simulink model "sampleModel2089"  (R2023a)
settings: Solver=VariableStepAuto  StartTime=0.0  StopTime=10.0  RelTol=1e-3
libraries: hdlsllib x3, simulink x3
settings Model: Creator=user1  LastModifiedBy=user1

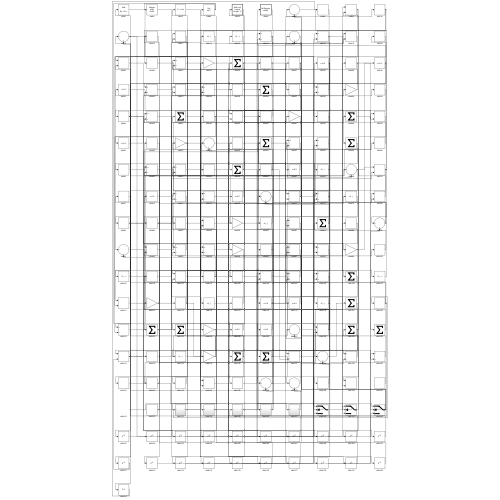
[thumbnail: Simulink's stored preview of the top-level diagram]
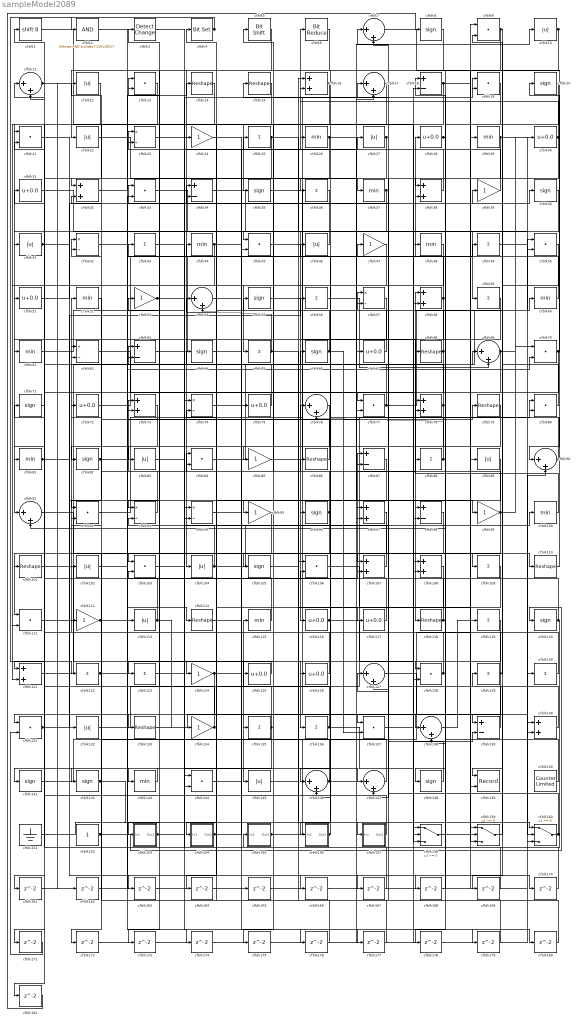
== system sampleModel2089 ==
  cfblk1 : ArithShift  BitShiftNumber=8
  cfblk{10,12,22,27,41,46,83,89,102,104,113,132,145} (13 alike) : Abs  SaturateOnIntegerOverflow=off
  cfblk{26,29,37,44,48,52,60..61,81,100,115,143} (12 alike) : MinMax
  cfblk{14..15,68,79,86,101,110,114,118,133} (10 alike) : Reshape
  cfblk{9,13,19,21,33,45,50,70,77,80,84,92,103,106,111,128,131,137,144} (19 alike) : DotProduct  OutDataTypeStr=Inherit: Inherit via internal rule
  cfblk{8,20,35,40,55,64,66,71,82,96,105,120,141..142,148} (15 alike) : Signum
  cfblk{16,32,38,58,73,78,97,107..108,121,140} (11 alike) : Sum
  cfblk{25,36,43,49,56,59,65,88,109,119,122..123,129..130,135..136} (16 alike) : Sum  Inputs=+
  cfblk{7,11,17,54,69,76,90..91,127,138,146..147} (12 alike) : Sum  Inputs=|++
  cfblk{24,39,47,53,85,95,99,112,124,134} (10 alike) : Gain
  cfblk{28,30..31,51,67,72,75,116..117,125..126} (11 alike) : Bias  Bias=0.0  SaturateOnIntegerOverflow=off
  cfblk{18,34,63,87,98,139} (6 alike) : Sum  Inputs=+-
  cfblk149 : Record  FileSettingsInternal="{\"entries\":[{\"content\":{\"excelSettings\":{\"content\":{},\"type\":\"Streamout.ExcelSettings\"}},\"type\":\"Streamout.FileSettingStorage\",\"uuid\":\"\"}],\"packageUris\":[\"http:\\/\\/schema.mathworks.com\\/mf0\\/streamout_blocks\\/R2020a\"],\"version\":\"1.0\"}"  Layout=[1 1]  SignalsInternal="{\"entries\":[{\"content\":{\"signals\":[{\"content\":{\"blockPath\":[],\"dimensions\":[1],\"domain\":\"\",\"lineColor\":\"#a2142f\",\"plots\":[1],\"port\":1,\"signalID\":6674,\"signalName\":\"XY Graph:1\"},\"type\":\"RecordBlkView.Signal\",\"uuid\":\"\"},{\"content\":{\"blockPath\":[],\"dimensions\":[1],\"domain\":\"\",\"lineColor\":\"#139fff\",\"plots\":[1],\"port\":2,\"signalID\":6677,\"signalName\":\"XY Graph:2\"},\"type\":\"RecordBlkView.Signal\",\"uuid\":\"\"}]},\"type\":\"RecordBlkView.InputSignals\",\"uuid\":\"\"}],\"packageUris\":[\"http:\\/\\/schema.mathworks.com\\/mf0\\/streamout_blocks\\/R2020a\"],\"version\":\"1.0\"}"  VisualizationBindings="{\"xyplotplugin\":{\"info\":[{\"series\":[{\"bindingParametersList\":[{\"parameter\":\"X-Axis\",\"signalID\":6674,\"signalName\":\"XY Graph:1\"},{\"parameter\":\"Y-Axis\",\"signalID\":6677,\"signalName\":\"XY Graph:2\"}],\"seriesID\":29365}],\"subplotID\":1}]}}"  CompatibilityTag=XY  st=-1
  cfblk150 : hdlsllib/Sources/Counter Limited  uplimit=7  tsamp=-1
  cfblk151 : Ground
  cfblk152 : Constant  SampleTime=-1
  cfblk153 : Subsystem
      settings: LibrarySourceBlock=|
      | hdlsllib/Ports &
      | Subsystems/Subsystem
  cfblk154 : Subsystem
      settings: LibrarySourceBlock=|
      | hdlsllib/Ports &
      | Subsystems/Subsystem
  cfblk155 : Subsystem
      settings: LibrarySourceBlock=|
      | hdlsllib/Ports &
      | Subsystems/Subsystem
  cfblk156 : Subsystem
      settings: LibrarySourceBlock=|
      | hdlsllib/Ports &
      | Subsystems/Subsystem
  cfblk157 : Subsystem
      settings: LibrarySourceBlock=|
      | hdlsllib/Ports &
      | Subsystems/Subsystem
  cfblk158 : Switch  SaturateOnIntegerOverflow=off  InputSameDT=off
  cfblk159 : Switch  SaturateOnIntegerOverflow=off  InputSameDT=off
  cfblk160 : Switch  SaturateOnIntegerOverflow=off  InputSameDT=off
  cfblk{161..181} (21 alike) : Delay  SampleTime=1
  cfblk2 : simulink/Logic and Bit Operations/Bitwise Operator  logicop=AND  UseBitMask=on  BitMask=bin2dec('11011001')  BitMaskRealWorld=Stored Integer
      settings: LibrarySourceBlock=|
      | hdlsllib/Logic and Bit
      | Operations/Bitwise
      | Operator
  cfblk{23,42,57,62,74,93..94} (7 alike) : Product  Inputs=*/  RndMeth=Zero  SaturateOnIntegerOverflow=on
  cfblk3 : simulink/Logic and Bit Operations/Detect Change  vinit=0  OutDataTypeStr=boolean
      settings: LibrarySourceBlock=|
      | hdlsllib/Logic and Bit
      | Operations/Detect
      | Change
  cfblk4 : simulink/Logic and Bit Operations/Bit Set  iBit=0
      settings: LibrarySourceBlock=|
      | hdlsllib/Logic and Bit
      | Operations/Bit Set
  cfblk5 : hdlsllib/Logic and Bit Operations/Bit Shift  mode=Shift Left Logical  N=0
  cfblk6 : hdlsllib/Logic and Bit Operations/Bit Reduce  mode=AND
  wires:
  cfblk46/1 -> cfblk45/1
  cfblk125/1 -> cfblk123/1
  cfblk38/1 -> cfblk6/1
  cfblk20/1 -> cfblk131/1
  cfblk5/1 -> cfblk104/1
  cfblk136/1 -> cfblk84/1, cfblk158/3
  cfblk47/1 -> cfblk65/1
  cfblk131/1 -> cfblk132/1, cfblk56/1
  cfblk99/1 -> cfblk103/1, cfblk70/1, cfblk72/1
  cfblk7/1 -> cfblk90/1
  cfblk72/1 -> cfblk44/1
  cfblk84/1 -> cfblk60/1
  cfblk138/1 -> cfblk119/1
  cfblk100/1 -> cfblk58/1
  cfblk80/1 -> cfblk57/1
  cfblk143/1 -> cfblk141/1
  cfblk14/1 -> cfblk91/1
  cfblk36/1 -> cfblk95/1
  cfblk97/1 -> cfblk143/1
  cfblk67/1 -> cfblk4/1
  cfblk123/1 -> cfblk74/1
  cfblk81/1 -> cfblk167/1, cfblk168/1
  cfblk8/1 -> cfblk22/1
  cfblk58/1 -> cfblk118/1, cfblk7/2
  cfblk19/1 -> cfblk98/1
  cfblk121/1 -> cfblk69/1
  cfblk142/1 -> cfblk160/1, cfblk112/1
  cfblk128/1 -> cfblk13/1, cfblk86/1, cfblk53/1
  cfblk126/1 -> cfblk52/1
  cfblk120/1 -> cfblk155/1(In1), cfblk76/1, cfblk93/2
  cfblk133/1 -> cfblk139/1
  cfblk107/1 -> cfblk34/1
  cfblk56/1 -> cfblk69/2
  cfblk88/1 -> cfblk55/1, cfblk76/2
  cfblk39/1 -> cfblk3/1
  cfblk4/1 -> cfblk122/1, cfblk2/1
  cfblk70/1 -> cfblk20/1, cfblk137/1
  cfblk95/1 -> cfblk111/1
  cfblk63/1 -> cfblk28/1
  cfblk40/1 -> cfblk41/1
  cfblk148/1 -> cfblk7/1
  cfblk15/1 -> cfblk21/1
  cfblk16/1 -> cfblk154/1(In1), cfblk111/2
  cfblk150/1 -> cfblk91/2
  cfblk93/1 -> cfblk73/1
  cfblk147/1 -> cfblk42/1
  cfblk41/1 -> cfblk99/1, cfblk163/1
  cfblk92/1 -> cfblk40/1
  cfblk90/1 -> cfblk18/1, cfblk63/2
  cfblk139/1 -> cfblk15/1
  cfblk158/1 -> cfblk89/1
  cfblk119/1 -> cfblk136/1
  cfblk155/1(Out1) -> cfblk29/1, cfblk107/2
  cfblk85/1 -> cfblk19/1
  cfblk132/1 -> cfblk80/1
  cfblk124/1 -> cfblk170/1, cfblk171/1
  cfblk111/1 -> cfblk64/1
  cfblk69/1 -> cfblk101/1, cfblk30/1
  cfblk104/1 -> cfblk9/1, cfblk13/2
  cfblk117/1 -> cfblk87/1
  cfblk55/1 -> cfblk138/1
  cfblk9/1 -> cfblk149/1, cfblk38/1
  cfblk61/1 -> cfblk24/1
  cfblk34/1 -> cfblk116/1
  cfblk129/1 -> cfblk145/1, cfblk144/2, cfblk11/2, cfblk9/2
  cfblk157/1(Out1) -> cfblk21/2
  cfblk152/1 -> cfblk120/1, cfblk62/1
  cfblk83/1 -> cfblk19/2
  cfblk140/1 -> cfblk33/1
  cfblk57/1 -> cfblk94/2
  cfblk159/1 -> cfblk129/1
  cfblk30/1 -> cfblk77/1, cfblk16/2, cfblk146/2
  cfblk96/1 -> cfblk5/1, cfblk173/1
  cfblk31/1 -> cfblk59/1
  cfblk43/1 -> cfblk105/1
  cfblk87/1 -> cfblk146/1
  cfblk73/1 -> cfblk83/1
  cfblk115/1 -> cfblk54/1
  cfblk94/1 -> cfblk79/1
  cfblk22/1 -> cfblk75/1
  cfblk141/1 -> cfblk39/1
  cfblk12/1 -> cfblk61/1
  cfblk110/1 -> cfblk80/2
  cfblk23/1 -> cfblk147/1
  cfblk156/1(Out1) -> cfblk66/1, cfblk46/1
  cfblk101/1 -> cfblk135/1
  cfblk37/1 -> cfblk45/2, cfblk175/1
  cfblk153/1(Out1) -> cfblk27/1, cfblk176/1
  cfblk2/1 -> cfblk114/1
  cfblk127/1 -> cfblk140/2
  cfblk76/1 -> cfblk133/1
  cfblk78/1 -> cfblk63/1, cfblk87/2
  cfblk154/1(Out1) -> cfblk47/1, cfblk179/1
  cfblk18/1 -> cfblk35/1, cfblk110/1
  cfblk160/1 -> cfblk43/1, cfblk62/2, cfblk78/2
  cfblk74/1 -> cfblk126/1
  cfblk71/1 -> cfblk121/1
  cfblk29/1 -> cfblk160/2, cfblk147/2
  cfblk79/1 -> cfblk82/1
  cfblk33/1 -> cfblk67/1
  cfblk113/1 -> cfblk102/1, cfblk134/1
  cfblk122/1 -> cfblk106/2, cfblk70/2
  cfblk49/1 -> cfblk130/1
  cfblk116/1 -> cfblk158/1, cfblk10/1
  cfblk105/1 -> cfblk117/1
  cfblk26/1 -> cfblk98/2, cfblk36/1
  cfblk77/1 -> cfblk50/1, cfblk23/2
  cfblk89/1 -> cfblk124/1
  cfblk137/1 -> cfblk139/2
  cfblk103/1 -> cfblk97/1
  cfblk112/1 -> cfblk42/2, cfblk38/2
  cfblk3/1 -> cfblk109/1
  cfblk6/1 -> cfblk93/1
  cfblk135/1 -> cfblk115/1, cfblk142/1, cfblk84/2
  cfblk51/1 -> cfblk34/2
  cfblk108/1 -> cfblk127/2
  cfblk11/1 -> cfblk48/1, cfblk162/1
  cfblk75/1 -> cfblk31/1
  cfblk45/1 -> cfblk77/2
  cfblk151/1 -> cfblk159/2
  cfblk32/1 -> cfblk14/1
  cfblk60/1 -> cfblk25/1
  cfblk52/1 -> cfblk92/1
  cfblk21/1 -> cfblk96/1
  cfblk1/1 -> cfblk108/2
  cfblk27/1 -> cfblk51/1, cfblk73/2
  cfblk65/1 -> cfblk157/1(In1), cfblk54/2
  cfblk118/1 -> cfblk11/1, cfblk148/1
  cfblk35/1 -> cfblk68/1
  cfblk82/1 -> cfblk113/1, cfblk78/1
  cfblk130/1 -> cfblk97/2
  cfblk91/1 -> cfblk144/1
  cfblk106/1 -> cfblk159/3
  cfblk24/1 -> cfblk37/1
  cfblk53/1 -> cfblk153/1(In1), cfblk177/1
  cfblk86/1 -> cfblk12/1
  cfblk102/1 -> cfblk49/1
  cfblk10/1 -> cfblk149/2, cfblk156/1(In1)
  cfblk44/1 -> cfblk121/2, cfblk107/1
  cfblk17/1 -> cfblk125/1
  cfblk62/1 -> cfblk158/2
  cfblk68/1 -> cfblk17/1, cfblk85/1
  cfblk28/1 -> cfblk128/1, cfblk178/1
  cfblk114/1 -> cfblk26/1
  cfblk134/1 -> cfblk103/2, cfblk71/1
  cfblk66/1 -> cfblk23/1, cfblk137/2
  cfblk145/1 -> cfblk100/1
  cfblk13/1 -> cfblk32/1
  cfblk146/1 -> cfblk32/2, cfblk88/1
  cfblk25/1 -> cfblk81/1, cfblk50/2
  cfblk48/1 -> cfblk161/1
  cfblk161/1 -> cfblk106/1
  cfblk162/1 -> cfblk33/2
  cfblk163/1 -> cfblk159/1
  cfblk109/1 -> cfblk164/1
  cfblk164/1 -> cfblk58/2
  cfblk54/1 -> cfblk165/1
  cfblk165/1 -> cfblk108/1
  cfblk144/1 -> cfblk166/1
  cfblk166/1 -> cfblk140/1
  cfblk167/1 -> cfblk94/1
  cfblk168/1 -> cfblk138/2
  cfblk50/1 -> cfblk169/1
  cfblk169/1 -> cfblk1/1
  cfblk170/1 -> cfblk57/2
  cfblk171/1 -> cfblk131/2
  cfblk98/1 -> cfblk172/1
  cfblk172/1 -> cfblk18/2
  cfblk173/1 -> cfblk17/2
  cfblk42/1 -> cfblk174/1
  cfblk174/1 -> cfblk90/2
  cfblk175/1 -> cfblk128/2
  cfblk176/1 -> cfblk74/2
  cfblk177/1 -> cfblk92/2
  cfblk178/1 -> cfblk160/3
  cfblk179/1 -> cfblk127/1
  cfblk64/1 -> cfblk180/1
  cfblk180/1 -> cfblk16/1
  cfblk59/1 -> cfblk181/1
  cfblk181/1 -> cfblk8/1

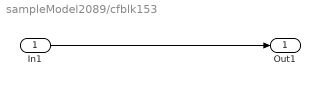
== system sampleModel2089/cfblk153 ==
  In1 : Inport
  Out1 : Outport
  wires:
  In1/1 -> Out1/1

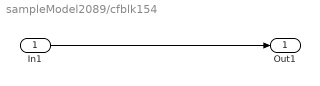
== system sampleModel2089/cfblk154 ==
  In1 : Inport
  Out1 : Outport
  wires:
  In1/1 -> Out1/1

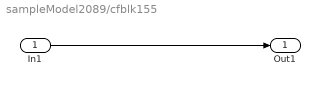
== system sampleModel2089/cfblk155 ==
  In1 : Inport
  Out1 : Outport
  wires:
  In1/1 -> Out1/1

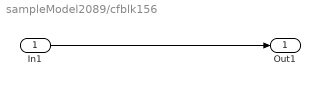
== system sampleModel2089/cfblk156 ==
  In1 : Inport
  Out1 : Outport
  wires:
  In1/1 -> Out1/1

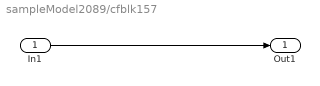
== system sampleModel2089/cfblk157 ==
  In1 : Inport
  Out1 : Outport
  wires:
  In1/1 -> Out1/1
